simulink model "ctlsea"  (R2021a)
settings: Solver=ode45  StartTime=0.0  StopTime=20  RelTol=1e-6  AbsTol=1e-6  EnableMultiTasking=on
InitFcn:
  | Ts=50e-3;
StopFcn:
  | epex219
libraries: spsSeriesRLCBranchLib x3, spsSampleandHoldLib x2, spsGroundLib x1, spspowerguiLib x1, spsControlledCurrentSourceLib x1, spsVoltageMeasurementLib x1
settings Model: Creator=amnlima  LastModifiedBy=dbnun
settings SolverCC: AutoScaleAbsTol=off  AlgebraicLoopSolver=TrustRegion
settings DataIOCC: LimitDataPoints=on  SaveFormat=Array  ReturnWorkspaceOutputs=off
settings OptimizationCC: LifeSpan=inf
settings DebuggingCC: SolverPrmCheckMsg=warning  AllowSymbolicDim=off  SFUnexpectedBacktrackingDiag=warning  SFNoUnconditionalDefaultTransitionDiag=warning  SFExecutionAtInitializationDiag=none  SFMachineParentedDataDiag=warning  ArithmeticOperatorsInVariantConditions=warning
settings HardwareCC: ProdBitPerPointer=32  ProdBitPerSizeT=32  ProdBitPerPtrDiffT=32  ProdLargestAtomicFloat=None  ProdIntDivRoundTo=Undefined  ProdEndianess=Unspecified  ProdWordSize=32  ProdHWDeviceType=32-bit Generic
settings ModelReferenceCC: PropagateSignalLabelsOutOfModel=off
settings SFSimCC: SimUseLocalCustomCode=off  CustomCodeUndefinedFunction=UseInterfaceOnly
settings RTWCC: RTWUseLocalCustomCode=off
settings CodeAppCC: StateflowObjectComments=on
settings GRTTargetCC: TargetLangStandard=C89/C90 (ANSI)
settings ConfigComp: CovMetricSettings=dw  CovSaveCumulativeToWorkspaceVar=on  CovSaveSingleToWorkspaceVar=on  CovExternalEMLEnable=off  CovSFcnEnable=off
settings SimscapeCC: SimscapeNormalizeSystem=off

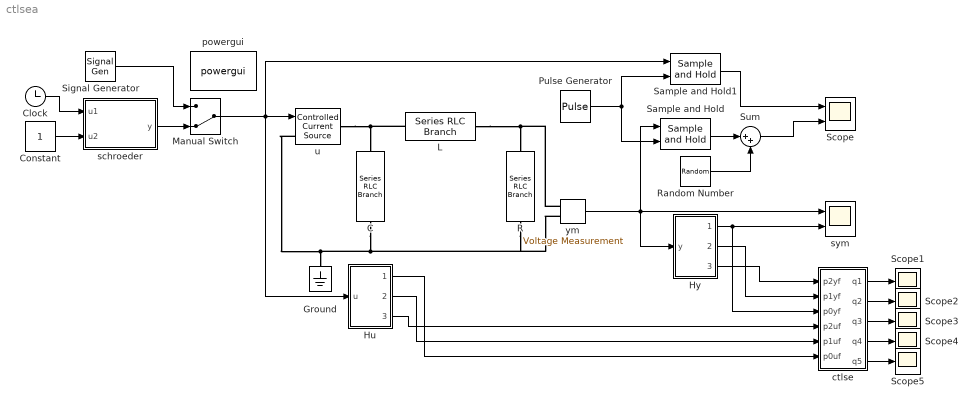
== system ctlsea ==
  C : spsSeriesRLCBranchLib/Series RLC Branch  LConnTagsString=__new0  RConnTagsString=__new0  BranchType=C  Resistance=1  Inductance=1e-3  SetiL0=off  InitialCurrent=0  Capacitance=1  Setx0=off  InitialVoltage=0  Measurements=None
  Clock : Clock
  Constant : Constant  SampleTime=-1
  Ground : spsGroundLib/Ground  LConnTagsString=a
  Hu : Subsystem
  Hy : Subsystem
  L : spsSeriesRLCBranchLib/Series RLC Branch  LConnTagsString=__new0  RConnTagsString=__new0  BranchType=L  Resistance=1  Inductance=1  SetiL0=off  InitialCurrent=0  Capacitance=1e-6  Setx0=off  InitialVoltage=0  Measurements=None
  Manual Switch : ManualSwitch  CurrentSetting=0
  Pulse Generator : DiscretePulseGenerator  PulseType=Time based  Period=Ts
  R : spsSeriesRLCBranchLib/Series RLC Branch  LConnTagsString=__new0  RConnTagsString=__new0  BranchType=R  Resistance=1  Inductance=1e-3  SetiL0=off  InitialCurrent=0  Capacitance=1e-6  Setx0=off  InitialVoltage=0  Measurements=None
  Random Number : RandomNumber  Variance=0  SampleTime=Ts
  Sample and Hold : spsSampleandHoldLib/Sample and Hold  ic=0  Ts=Ts
      settings: SourceProductBaseCode=PS
  Sample and Hold1 : spsSampleandHoldLib/Sample and Hold  ic=0  Ts=Ts
      settings: SourceProductBaseCode=PS
  Scope : Scope  NumInputPorts=2
  Scope{1..5} (5 alike) : Scope
  Signal Generator : SignalGenerator  WaveForm=sawtooth  Units=rad/sec
  Sum : Sum  Inputs=|++
  ctlse : Subsystem
  powergui : spspowerguiLib/powergui  Priority=1  SimulationMode=Continuous  SampleTime=50e-6  frequency=60  Iterations=50  frequencyindice=0  Pbase=100e6  ErrMax=1e-4  UnitsV=kV  UnitsW=MW  buscounter=0  FunctionMessages=off  echomessages=off  EnableUseOfTLC=off  CurrentSourceSwitches=on  DisableSnubberDevices=off  DisableRonSwitches=off  DisableVfSwitches=off  DisplayEquations=off  AutomaticDiscreteSolvers=off  SolverType=Tustin  Interpol=off  ExternalGateDelay=off  methode=off  Ts=0  x0status=zero  SPID=off  SwTol=0  HookPort=off  NonlinearTolerance=1e-4  nMaxIteration=100  ContinueOnMaxIteration=off  RestoreLinks=warning  ResistiveCurrentMeasurement=off  Frange=[0:2:500]  Ylog=off  Xlog=on  ShowGrid=off  save=off  variable=ZData  structure=0  ZoomFFT=off  StartTime=0.0  cycles=1  DisplayStyle=1  fundamental=60  FreqAxis=off  MaxFrequency=1000  frequencyindicesteady=1  RmsSteady=1  display=off
  schroeder : MATLAB Function  TreatAsAtomicUnit=on
      settings: AttributesFormatString=%<SystemSampleTime>
  sym : Scope  NumInputPorts=2
  u : spsControlledCurrentSourceLib/Controlled Current Source  Initialize=on  Source_Type=AC  Amplitude=0  Phase=0  Frequency=0  Measurements=None
  ym : spsVoltageMeasurementLib/Voltage Measurement  PhasorSimulation=off  OutputType=Complex  PSBequivalent=0
  wires:
  ym/1 -> Hy/1(y), sym/1, Sample and Hold/1
  Pulse Generator/1 -> Sample and Hold1/2, Sample and Hold/2
  Sample and Hold1/1 -> Scope/1
  Clock/1 -> schroeder/1(u1)
  Constant/1 -> schroeder/2(u2)
  ctlse/1(q1) -> Scope1/1
  ctlse/2(q2) -> Scope2/1
  ctlse/3(q3) -> Scope3/1
  ctlse/4(q4) -> Scope4/1
  Sample and Hold/1 -> Sum/1
  Random Number/1 -> Sum/2
  Sum/1 -> Scope/2
  ctlse/5(q5) -> Scope5/1
  Manual Switch/1 -> Hu/1(u), Sample and Hold1/1, u/1
  Signal Generator/1 -> Manual Switch/1
  schroeder/1(y) -> Manual Switch/2
  Hy/1(p0yf) -> ctlse/3(p0yf), sym/2
  Hy/3(p2yf) -> ctlse/1(p2yf)
  Hy/2(p1yf) -> ctlse/2(p1yf)
  Hu/3(p2uf) -> ctlse/4(p2uf)
  Hu/2(p1uf) -> ctlse/5(p1uf)
  Hu/1(p0uf) -> ctlse/6(p0uf)
  connections:
  R/RConn1 -- ym/LConn2 -- C/RConn1 -- Ground/LConn1 -- u/LConn1
  L/LConn1 -- C/LConn1 -- u/RConn1
  L/RConn1 -- R/LConn1 -- ym/LConn1

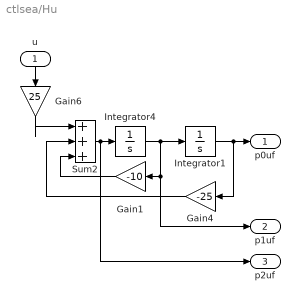
== system ctlsea/Hu ==
  u : Inport
  Gain1 : Gain  Gain=-10
  Gain4 : Gain  Gain=-25
  Gain6 : Gain  Gain=25
  Integrator1 : Integrator
  Integrator4 : Integrator
  Sum2 : Sum  Inputs=|+++
  p0uf : Outport  VectorParamsAs1DForOutWhenUnconnected=off
  p1uf : Outport  Port=2  VectorParamsAs1DForOutWhenUnconnected=off
  p2uf : Outport  Port=3  VectorParamsAs1DForOutWhenUnconnected=off
  wires:
  u/1 -> Gain6/1
  Integrator1/1 -> Gain4/1, p0uf/1
  Sum2/1 -> p2uf/1, Integrator4/1
  Gain1/1 -> Sum2/3
  Integrator4/1 -> Integrator1/1, p1uf/1, Gain1/1
  Gain6/1 -> Sum2/1
  Gain4/1 -> Sum2/2

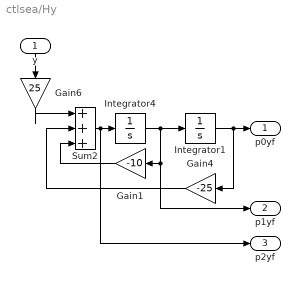
== system ctlsea/Hy ==
  y : Inport
  Gain1 : Gain  Gain=-10
  Gain4 : Gain  Gain=-25
  Gain6 : Gain  Gain=25
  Integrator1 : Integrator
  Integrator4 : Integrator
  Sum2 : Sum  Inputs=|+++
  p0yf : Outport  VectorParamsAs1DForOutWhenUnconnected=off
  p1yf : Outport  Port=2  VectorParamsAs1DForOutWhenUnconnected=off
  p2yf : Outport  Port=3  VectorParamsAs1DForOutWhenUnconnected=off
  wires:
  y/1 -> Gain6/1
  Integrator1/1 -> Gain4/1, p0yf/1
  Sum2/1 -> p2yf/1, Integrator4/1
  Gain1/1 -> Sum2/3
  Integrator4/1 -> Integrator1/1, p1yf/1, Gain1/1
  Gain6/1 -> Sum2/1
  Gain4/1 -> Sum2/2

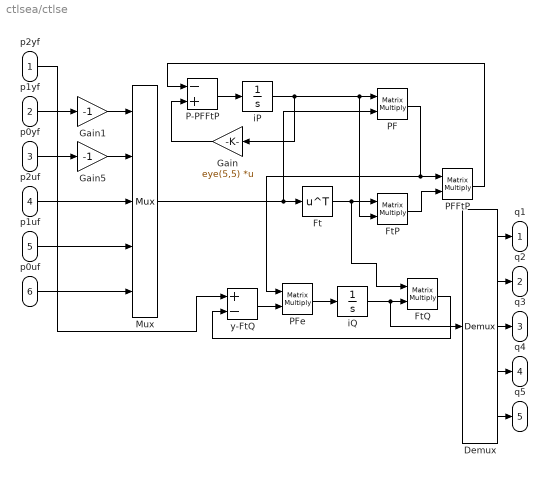
== system ctlsea/ctlse ==
  p2yf : Inport
  p1yf : Inport  Port=2
  p0yf : Inport  Port=3
  p2uf : Inport  Port=4
  p1uf : Inport  Port=5
  p0uf : Inport  Port=6
  Demux : Demux  Outputs=5
      settings: DisplayOption=none
  Ft : Math  Operator=transpose  SignedPower=on  SaturateOnIntegerOverflow=on
  FtP : Product  Multiplication=Matrix(*)
  FtQ : Product  Multiplication=Matrix(*)
  Gain : Gain  Gain=eye(5,5)  Multiplication=Matrix(K*u)
  Gain1 : Gain  Gain=-1
  Gain5 : Gain  Gain=-1
  Mux : Mux  Inputs=5
  P-PFFtP : Sum  Inputs=-+
  PF : Product  Multiplication=Matrix(*)
  PFFtP : Product  Multiplication=Matrix(*)
  PFe : Product  Multiplication=Matrix(*)
  iP : Integrator  InitialCondition=1e3*eye(5,5)
  iQ : Integrator  InitialCondition=zeros(5,1)
  y-FtQ : Sum  Inputs=+-
  q1 : Outport  VectorParamsAs1DForOutWhenUnconnected=off
  q2 : Outport  Port=2  VectorParamsAs1DForOutWhenUnconnected=off
  q3 : Outport  Port=3  VectorParamsAs1DForOutWhenUnconnected=off
  q4 : Outport  Port=4  VectorParamsAs1DForOutWhenUnconnected=off
  q5 : Outport  Port=5  VectorParamsAs1DForOutWhenUnconnected=off
  wires:
  P-PFFtP/1 -> iP/1
  Gain/1 -> P-PFFtP/2
  Mux/1 -> Ft/1, PF/2
  PF/1 -> PFFtP/1, PFe/1
  FtP/1 -> PFFtP/2
  Ft/1 -> FtP/1, FtQ/1
  iQ/1 -> Demux/1, FtQ/2
  FtQ/1 -> y-FtQ/2
  PFe/1 -> iQ/1
  y-FtQ/1 -> PFe/2
  Gain1/1 -> Mux/1
  Gain5/1 -> Mux/2
  Demux/1 -> q1/1
  iP/1 -> Gain/1, FtP/2, PF/1
  Demux/2 -> q2/1
  Demux/3 -> q3/1
  Demux/4 -> q4/1
  Demux/5 -> q5/1
  PFFtP/1 -> P-PFFtP/1
  p2yf/1 -> y-FtQ/1
  p1yf/1 -> Gain1/1
  p0yf/1 -> Gain5/1
  p2uf/1 -> Mux/3
  p1uf/1 -> Mux/4
  p0uf/1 -> Mux/5

== matlab function ctlsea/schroeder ==
  settings: updateMethod=DISCRETE
  data: u1 input; y output; u2 input
function y = fcn(u1,u2)
%#codegen
t=u1;
s=u2;
%
fmin=1/2/pi;fmax=1/pi;etaf=(fmax-fmin)/16;
fk=(fmin:etaf:fmax)';
N=length(fk);
ak=1.0*ones(size(fk));
pk=-[(1:N).*(0:N-1)]'*(pi/N);
tmp=0*(1:N);
y=0;
if s==0,
    y=asin(sin(t));
elseif s==1,
    for i=1:N,
        tmp(i)=ak(i)*cos(2*pi*fk(i)*t+pk(i));
    end
    y=sum(tmp);
elseif s==2,
    y=rand();
else
    y=sin(t);
end
